simulink model "throttleTest"  (R2021b)
settings: Solver=VariableStepAuto  StartTime=0.0  StopTime=20  RelTol=1e-3
libraries: aerolibanimutils x3
settings Model: Creator=Aidan  LastModifiedBy=Aidan

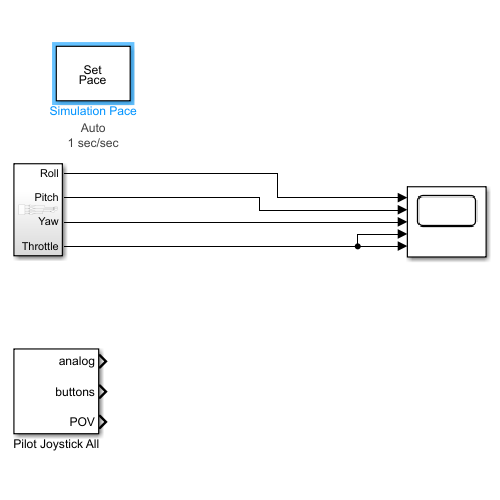
[thumbnail: Simulink's stored preview of the top-level diagram]
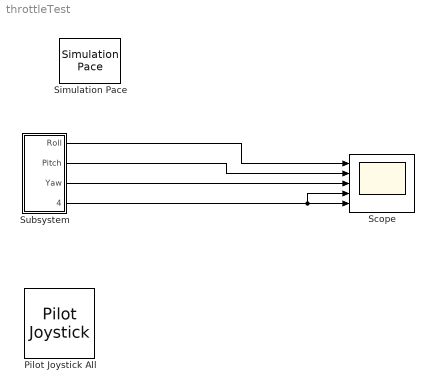
== system throttleTest ==
  Pilot Joystick All : aerolibanimutils/Pilot Joystick  JoystickID=Joystick1  OutputConfiguration=AllOutputs  SampleTime=1/30
  Scope : Scope  NumInputPorts=5
  Simulation Pace : aerolibanimutils/Simulation Pace  SimulationPace=1  SleepMode=Auto  OutputPaceError=off  SampleTime=1/30
  Subsystem : Subsystem
  wires:
  Subsystem/4(Throttle) -> Scope/5, Scope/4
  Subsystem/1(Roll) -> Scope/1
  Subsystem/2(Pitch) -> Scope/2
  Subsystem/3(Yaw) -> Scope/3

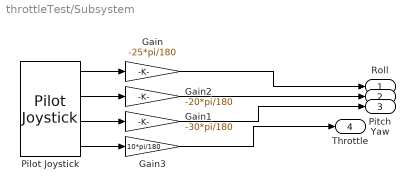
== system throttleTest/Subsystem ==
  Gain : Gain  Gain=-25*pi/180
  Gain1 : Gain  Gain=-30*pi/180
  Gain2 : Gain  Gain=-20*pi/180
  Gain3 : Gain  Gain=10*pi/180
  Pilot Joystick : aerolibanimutils/Pilot Joystick  JoystickID=Joystick1  OutputConfiguration=FourAxis  SampleTime=1/30
  Roll : Outport
  Pitch : Outport  Port=2
  Yaw : Outport  Port=3
  Throttle : Outport  Port=4
  wires:
  Pilot Joystick/2 -> Gain2/1
  Pilot Joystick/3 -> Gain1/1
  Gain2/1 -> Pitch/1
  Pilot Joystick/1 -> Gain/1
  Gain/1 -> Roll/1
  Pilot Joystick/4 -> Gain3/1
  Gain3/1 -> Throttle/1
  Gain1/1 -> Yaw/1
